simulink model "KP_01"  (R2018a)
settings: Solver=FixedStepAuto  StartTime=0.0  StopTime=5  FixedStep=1e-3  RelTol=1e-3
undefined symbols (not defined in the file or in its folder): now
libraries: sl_kafka_lib x2
settings Model: Creator=asolland  LastModifiedBy=asolland
settings OptimizationCC: DefaultParameterBehavior=Inlined  EnhancedBackFolding=on  PassReuseOutputArgsAs=Individual arguments  OptimizeBlockOrder=speed  DifferentSizesBufferReuse=on  OptimizationCustomize=off
settings DebuggingCC: ParameterTunabilityLossMsg=error
settings HardwareCC: ProdLongLongMode=on
settings SFSimCC: SimUseLocalCustomCode=on  MATLABDynamicMemAlloc=off
settings RTWCC: Description=Kafka Target  SystemTargetFile=kafkatarget.tlc  TemplateMakefile=ert_default_tmf  GenerateReport=on  RTWUseLocalCustomCode=on  IncludeHyperlinkInReport=on  GenerateTraceInfo=on  GenerateTraceReport=on  GenerateTraceReportSl=on  GenerateTraceReportSf=on  GenerateTraceReportEml=on
settings CodeAppCC: ForceParamTrailComments=on  IgnoreCustomStorageClasses=off  OperatorAnnotations=on  SimulinkDataObjDesc=on  SFDataObjDesc=on  InsertBlockDesc=on
settings STFCustomTargetCC: TargetLangStandard=C99 (ISO)  MultiwordLength=256  GenerateSampleERTMain=on  CombineOutputUpdateFcns=on  ERTCustomFileBanners=on  SupportContinuousTime=off  SupportNonInlinedSFcns=off  RemoveResetFunc=on  MATLABClassNameForMDSCustomization=Simulink.SoftwareTarget.ERTCustomization  GRTInterface=off  UseToolchainInfoCompliant=on  SystemTargetFile=kafkatarget.tlc
settings ERTTargetCC: TargetLangStandard=C99 (ISO)  GenerateSampleERTMain=on  ParMdlRefBuildCompliant=off  CompOptLevelCompliant=off  ConcurrentExecutionCompliant=off  ModelStepFunctionPrototypeControlCompliant=off  CPPClassGenCompliant=off  InlinedParameterPlacement=NonHierarchical  ERTCustomFileTemplate=kafkatarget_process.tlc

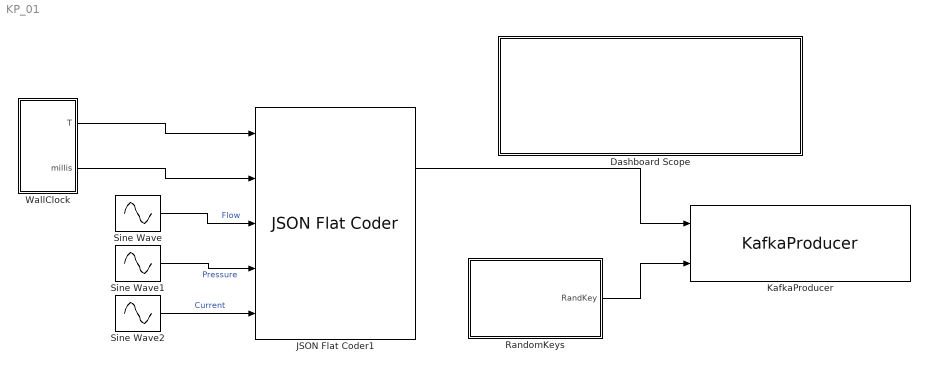
== system KP_01 ==
  Dashboard Scope : Subsystem  DialogController=hmiCreateDDGDialog  IsWebBlock=on  mask(MWDashboardBlock){webBlockId=2e5dd33c-565c-4a22-b828-7506f52d7db4, webBlockType=sdiscope, ShowInLibBrowser=on, ShowInitialText=on, HMISrcModelName=KP_01}
      mask prompts: webBlockId "WebBlock Id"; webBlockType "WebBlock Type"; HMISrcModelName "Source Model"
      mask help: Traces signals on the dashboard scope during simulation.
      mask Help: helpview([docroot '/mapfiles/simulink.map'], 'hmi_scope')
      mask Display:
      | if strcmp(get_param(bdroot(gcb),'BlockDiagramType'),'library')
      |  image([(matlabroot) '/toolbox/simulink/hmi/icons/SDIScope.png'])
      | end
  JSON Flat Coder1 : sl_kafka_lib/JSON Flat Coder  sfpDirection=Encode  sfpLength=200  sfpFields={'TS', 'M', 'Flow', 'Pressure', 'Current'}  sfpOutLength=on  sfpInLength=on
      settings: SourceProductName=Kafka Library
  KafkaProducer : sl_kafka_lib/KafkaProducer  sfpBrokers='localhost:9092'  sfpTopic='sltopic'  sfpKeyAsInput=on  sfpKeyAsInputLen=32  sfpKey='mykey'  sfpMsgLen=200  sfpTS=.1  sfpExtTimestamp=off  sfpConf=|  sfpTopicConf=compression.level=-1
      | client.id=sl_kafka_producer
      | message.copy.max.bytes=65535
      settings: SourceProductName=Kafka Library
  RandomKeys : Subsystem
  Sine Wave : Sin  SineType=Sample based  Amplitude=15  Bias=20  Samples=100  SampleTime=0.02  Offset=88
  Sine Wave1 : Sin  SineType=Sample based  Amplitude=20  Bias=30  Samples=100  SampleTime=0.05  Offset=20
  Sine Wave2 : Sin  SineType=Sample based  Amplitude=10  Bias=3  Samples=100  SampleTime=0.08  Offset=44
  WallClock : Subsystem
  wires:
  Sine Wave/1 -> JSON Flat Coder1/3  "Flow"
  Sine Wave1/1 -> JSON Flat Coder1/4  "Pressure"
  Sine Wave2/1 -> JSON Flat Coder1/5  "Current"
  JSON Flat Coder1/1 -> KafkaProducer/1
  WallClock/1(T) -> JSON Flat Coder1/1
  WallClock/2(millis) -> JSON Flat Coder1/2
  RandomKeys/1(RandKey) -> KafkaProducer/2

== system KP_01/Dashboard Scope ==

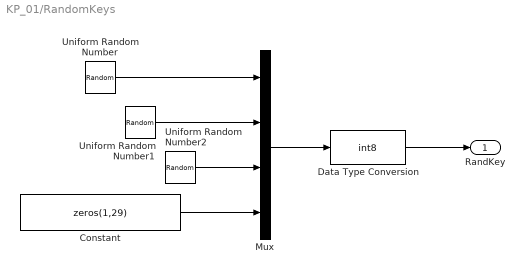
== system KP_01/RandomKeys ==
  Constant : Constant  Value=zeros(1,29)  OutDataTypeStr=double
  Data Type Conversion : DataTypeConversion  OutDataTypeStr=int8
  Mux : Mux
  Uniform Random Number : UniformRandomNumber  Minimum=65  Maximum=90  Seed=round(1000000*mod(now,1))  SampleTime=1e-3
  Uniform Random Number1 : UniformRandomNumber  Minimum=65  Maximum=90  Seed=round(2000000*mod(now,1))  SampleTime=1e-3
  Uniform Random Number2 : UniformRandomNumber  Minimum=65  Maximum=90  Seed=round(3000000*mod(now,1))  SampleTime=1e-3
  RandKey : Outport  VectorParamsAs1DForOutWhenUnconnected=off
  wires:
  Uniform Random Number/1 -> Mux/1
  Mux/1 -> Data Type Conversion/1
  Uniform Random Number1/1 -> Mux/2
  Uniform Random Number2/1 -> Mux/3
  Constant/1 -> Mux/4
  Data Type Conversion/1 -> RandKey/1

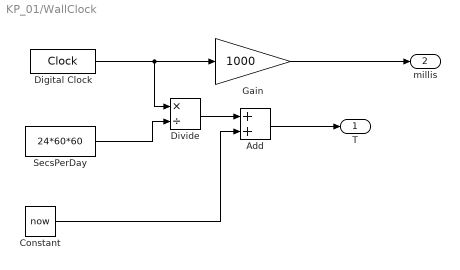
== system KP_01/WallClock ==
  Add : Sum
  Constant : Constant  Value=now
  Digital Clock : DigitalClock  SampleTime=1e-3
  Divide : Product  Inputs=*/
  Gain : Gain  Gain=1000
  SecsPerDay : Constant  Value=24*60*60
  T : Outport  VectorParamsAs1DForOutWhenUnconnected=off
  millis : Outport  Port=2  VectorParamsAs1DForOutWhenUnconnected=off
  wires:
  Add/1 -> T/1
  Divide/1 -> Add/1
  SecsPerDay/1 -> Divide/2
  Digital Clock/1 -> Divide/1, Gain/1
  Constant/1 -> Add/2
  Gain/1 -> millis/1
